simulink model "lab8_sl"  (R2021b)
settings: Solver=ode45  StartTime=0.0  StopTime=15.0  MaxStep=0.02  MinStep=0.01  RelTol=1e-3
settings Model: Creator=JaSzw  LastModifiedBy=JaSzw
settings SolverCC: InitialStep=0.01

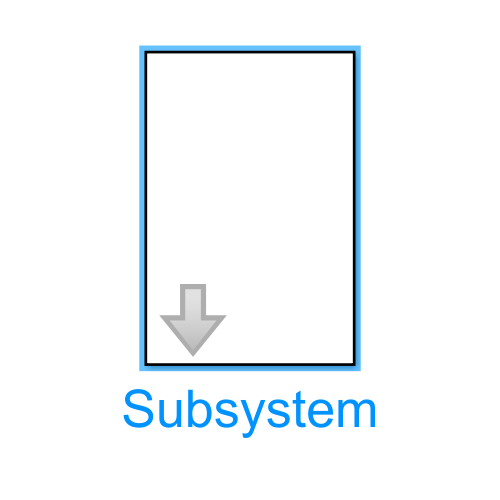
[thumbnail: Simulink's stored preview of the top-level diagram]
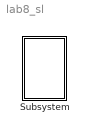
== system lab8_sl ==
  Subsystem : Subsystem  mask{n=3, g=9.81, k=1, m=2, l=4, x=-1, y=-1, xi=[-1 1 1], yi=[1 1 -1], di=[0.1 0.1 0.1], ai=[1 -1 1.5]}

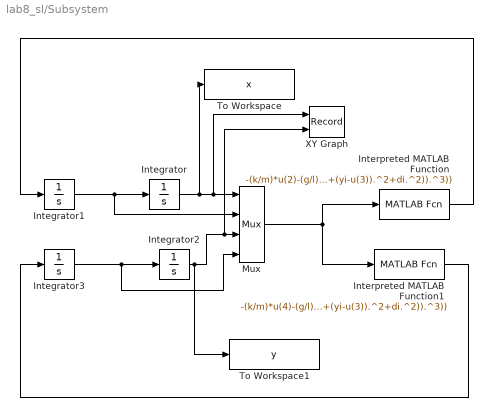
== system lab8_sl/Subsystem ==
  Integrator : Integrator  InitialCondition=-1
  Integrator1 : Integrator
  Integrator2 : Integrator  InitialCondition=-1
  Integrator3 : Integrator
  Interpreted MATLAB Function : MATLABFcn  MATLABFcn=-(k/m)*u(2)-(g/l)*u(1)+sum(ai.*((xi-u(1))./(sqrt((xi-u(1)).^2+(yi-u(3)).^2+di.^2)).^3))  OutputDimensions=1
  Interpreted MATLAB Function1 : MATLABFcn  MATLABFcn=-(k/m)*u(4)-(g/l)*u(3)+sum(ai.*((yi-u(3))./(sqrt((xi-u(1)).^2+(yi-u(3)).^2+di.^2)).^3))  OutputDimensions=1
  Mux : Mux
  To Workspace : ToWorkspace  VariableName=x  SampleTime=-1
  To Workspace1 : ToWorkspace  VariableName=y  SampleTime=-1
  XY Graph : Record  FileSettingsInternal="{\"entries\":[{\"content\":{\"excelSettings\":{\"content\":{},\"type\":\"Streamout.ExcelSettings\"}},\"type\":\"Streamout.FileSettingStorage\",\"uuid\":\"80bf781d-886b-4910-8d11-966c4393c2d9\"}],\"packageUris\":[\"http://schema.mathworks.com/mf0/streamout_blocks/R2020a\"],\"version\":\"1.0\"}"  Layout=[1 1]  SignalsInternal="{\"entries\":[{\"content\":{\"signals\":[{\"content\":{\"blockPath\":[\"untitled/XY Graph\"],\"channel\":[],\"dimensions\":[1],\"domain\":\"untitled/XY Graph\",\"lineColor\":\"#a2142f\",\"plots\":[1],\"port\":1,\"sid\":[],\"signalID\":25,\"signalName\":\"XY Graph:1\"},\"type\":\"RecordBlkView.Signal\",\"uuid\":\"91e320a5-2fba-48aa-a424-ca6bc039878b\"},{\"content\":{\"blockPath\":[\"untitled/XY Graph\"],\"channel\":[],\"dimensions\":[1],\"domain\":\"untitled/XY Graph\",\"lineColor\":\"#139fff\",\"plots\":[1],\"port\":2,\"sid\":[],\"signalID\":28,\"signalName\":\"XY Graph:2\"},\"type\":\"RecordBlkView.Signal\",\"uuid\":\"14643981-c5d7-4412-a3ef-a451edc3ee38\"}]},\"type\":\"RecordBlkView.InputSignals\",\"uuid\":\"fb35c58e-3930-4c22-9125-7e7b02b50d71\"}],\"packageUris\":[\"http://schema.mathworks.com/mf0/streamout_blocks/R2020a\"],\"version\":\"1.0\"}"  VisualizationBindings="{\"xyplotplugin\":{\"info\":[{\"series\":[{\"bindingParametersList\":[{\"parameter\":\"X-Axis\",\"signalID\":25,\"signalName\":\"XY Graph:1\"},{\"parameter\":\"Y-Axis\",\"signalID\":28,\"signalName\":\"XY Graph:2\"}],\"seriesID\":787}],\"subplotID\":1}]}}"  CompatibilityTag=XY
  wires:
  Interpreted MATLAB Function/1 -> Integrator1/1
  Integrator3/1 -> Mux/4, Integrator2/1
  Mux/1 -> Interpreted MATLAB Function1/1, Interpreted MATLAB Function/1
  Interpreted MATLAB Function1/1 -> Integrator3/1
  Integrator1/1 -> Mux/2, Integrator/1
  Integrator2/1 -> To Workspace1/1, XY Graph/2, Mux/3
  Integrator/1 -> To Workspace/1, XY Graph/1, Mux/1
